simulink model "Inductance_Scan_model"  (R2022a)
settings: Solver=FixedStepAuto  StartTime=0.0  StopTime=.004  FixedStep=SampleTime  RelTol=1e-3
values from neighbouring files (symbols this model uses):
  Ad = sys_d_plasma.A    [All_injectors_LQG_bop_plasma_ss_model_code.m]    (also in All_injectors_LQG_bop_ss_model_code.m; All_injectors_LQG_continuous_time_code.m; All_injectors_LQG_plasma_7_15_24_code.m; All_injectors_LQG_plasma_ss_model_code.m)
  Amplitude = 600    [All_injectors_LQG_bop_plasma_ss_model_code.m]    (also in All_injectors_LQG_bop_ss_model_code.m; All_injectors_LQG_continuous_time_code.m; All_injectors_LQG_plasma_7_15_24_code.m; All_injectors_LQG_plasma_ss_model_code.m)
  Amplitude1 = 600    [All_injectors_vaccum.m]    (also in All_injectors_with_LQG_code.m; MPC_attempt.m; Plasma_ss_model.m; Use_for_freq_scan.m)
  Bd = sys_d_plasma.B    [All_injectors_LQG_bop_plasma_ss_model_code.m]    (also in All_injectors_LQG_bop_ss_model_code.m; All_injectors_LQG_continuous_time_code.m; All_injectors_LQG_plasma_7_15_24_code.m; All_injectors_LQG_plasma_ss_model_code.m)
  Cap = 96e-6    (= 9.6e-05)    [All_injectors_LQG_bop_ss_model_code.m]    (also in All_injectors_LQG_continuous_time_code.m; All_injectors_LQG_plasma_7_15_24_code.m; All_injectors_LQG_plasma_ss_model_code.m; All_injectors_vaccum.m)
  Cd = sys_d_plasma.C    [All_injectors_LQG_bop_plasma_ss_model_code.m]    (also in All_injectors_LQG_bop_ss_model_code.m; All_injectors_LQG_continuous_time_code.m; All_injectors_LQG_plasma_7_15_24_code.m; All_injectors_LQG_plasma_ss_model_code.m)
  Dd = sys_d_plasma.D    [All_injectors_LQG_bop_plasma_ss_model_code.m]    (also in All_injectors_LQG_bop_ss_model_code.m; All_injectors_LQG_continuous_time_code.m; All_injectors_LQG_plasma_7_15_24_code.m; All_injectors_LQG_plasma_ss_model_code.m)
  L1 = (9.78e-7)    (= 9.78e-07)    [All_injectors_LQG_bop_plasma_ss_model_code.m]    (also in All_injectors_LQG_bop_ss_model_code.m = 8.0141e-07; All_injectors_LQG_continuous_time_code.m = 8.0141e-07; All_injectors_LQG_plasma_7_15_24_code.m = 8.0141e-07; All_injectors_LQG_plasma_ss_model_code.m = 8.0141e-07)
  L2 = 2.0462e-6    (= 2.0462e-06)    [All_injectors_LQG_bop_ss_model_code.m]    (also in All_injectors_LQG_continuous_time_code.m; All_injectors_LQG_plasma_7_15_24_code.m; All_injectors_LQG_plasma_ss_model_code.m; All_injectors_vaccum.m = 9.3369e-07)
  Lp = L2    (= 2.0462e-06)    [All_injectors_LQG_bop_ss_model_code.m]    (also in All_injectors_LQG_continuous_time_code.m; All_injectors_LQG_plasma_7_15_24_code.m; All_injectors_LQG_plasma_ss_model_code.m; Plasma_ss_model.m = 1.0231e-06)
  M = .161*L2    (= 3.294382e-07)    [All_injectors_LQG_bop_ss_model_code.m]    (also in All_injectors_LQG_continuous_time_code.m; All_injectors_LQG_plasma_7_15_24_code.m; All_injectors_LQG_plasma_ss_model_code.m; All_injectors_vaccum.m = 1.5032409e-07)
  Mw = .1346*L2    (= 2.7541852e-07)    [All_injectors_LQG_bop_ss_model_code.m]    (also in All_injectors_LQG_continuous_time_code.m; All_injectors_LQG_plasma_7_15_24_code.m; All_injectors_LQG_plasma_ss_model_code.m; All_injectors_vaccum.m = 1.25674674e-07)
  NoisePower = 0    [All_injectors_LQG_bop_plasma_ss_model_code.m]    (also in All_injectors_LQG_bop_ss_model_code.m = 0.0001; All_injectors_LQG_continuous_time_code.m = 0.0001; All_injectors_LQG_plasma_7_15_24_code.m; All_injectors_LQG_plasma_ss_model_code.m = 0.0001)
  R = 1    [All_injectors_LQG_bop_plasma_ss_model_code.m]    (also in All_injectors_LQG_bop_ss_model_code.m = diag(1*ones(1,num_inputs)); All_injectors_LQG_continuous_time_code.m = diag(1*ones(1,num_inputs)); All_injectors_LQG_plasma_7_15_24_code.m = diag(1*ones(1,num_inputs)); All_injectors_LQG_plasma_ss_model_code.m = diag(1*ones(1,num_inputs)))
  R1 = .0025    (= 0.0025)    [All_injectors_LQG_bop_ss_model_code.m]    (also in All_injectors_LQG_continuous_time_code.m; All_injectors_LQG_plasma_7_15_24_code.m; All_injectors_LQG_plasma_ss_model_code.m; All_injectors_vaccum.m)
  R2 = .005    (= 0.005)    [All_injectors_LQG_bop_ss_model_code.m]    (also in All_injectors_LQG_continuous_time_code.m; All_injectors_LQG_plasma_7_15_24_code.m; All_injectors_LQG_plasma_ss_model_code.m; All_injectors_vaccum.m)
  R3 = .005    (= 0.005)    [All_injectors_LQG_bop_ss_model_code.m]    (also in All_injectors_LQG_continuous_time_code.m; All_injectors_LQG_plasma_7_15_24_code.m; All_injectors_LQG_plasma_ss_model_code.m; All_injectors_vaccum.m)
  RunTime = .004    (= 0.004)    [All_injectors_LQG_bop_plasma_ss_model_code.m]    (also in All_injectors_LQG_bop_ss_model_code.m; All_injectors_LQG_continuous_time_code.m; All_injectors_LQG_plasma_7_15_24_code.m; All_injectors_LQG_plasma_ss_model_code.m)
  SampleTime = 1e-7    (= 1e-07)    [All_injectors_LQG_bop_plasma_ss_model_code.m]    (also in All_injectors_LQG_bop_ss_model_code.m; All_injectors_LQG_continuous_time_code.m; All_injectors_LQG_plasma_7_15_24_code.m; All_injectors_LQG_plasma_ss_model_code.m)
  voltage = Amplitude*sin(2*pi*Frequency*time)    [All_injectors_LQG_bop_plasma_ss_model_code.m]    (also in All_injectors_LQG_bop_ss_model_code.m; All_injectors_LQG_continuous_time_code.m; All_injectors_LQG_plasma_7_15_24_code.m; All_injectors_LQG_plasma_ss_model_code.m)
undefined symbols (not defined in the file or in its folder): Discrete, L1_V, Time
libraries: spsSeriesRLCBranchLib x50, simulink x23, spsCurrentMeasurementLib x20, spsDCVoltageSourceLib x12, spsVoltageMeasurementLib x11, spsFullBridgeMMCExternalDCLinksLib x9, spsPWMGeneratorMultilevelLib x9, ctrlSharedLib x5, spsMosfetLib x4, spsParallelRLCBranchLib x2, spsMutualInductanceLib x1, spspowerguiLib x1
(part 2 of 2)

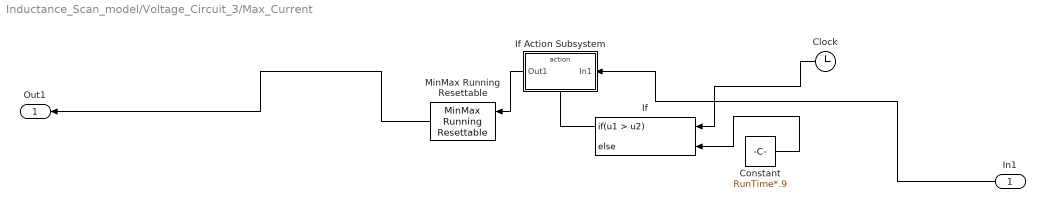
== system Inductance_Scan_model/Voltage_Circuit_3/Max_Current ==
  In1 : Inport
  Clock : Clock
  Constant : Constant  Value=RunTime*.9
  If : If  NumInputs=2  IfExpression=u1 > u2
  If Action Subsystem : Subsystem  TreatAsAtomicUnit=on
  MinMax Running Resettable : simulink/Math Operations/MinMax Running Resettable  Function=max  vinit=0.0
  Out1 : Outport
  wires:
  In1/1 -> If Action Subsystem/1(In1)
  If Action Subsystem/1(Out1) -> MinMax Running Resettable/1
  MinMax Running Resettable/1 -> Out1/1
  Constant/1 -> If/2
  Clock/1 -> If/1
  If/1 -> If Action Subsystem/Action

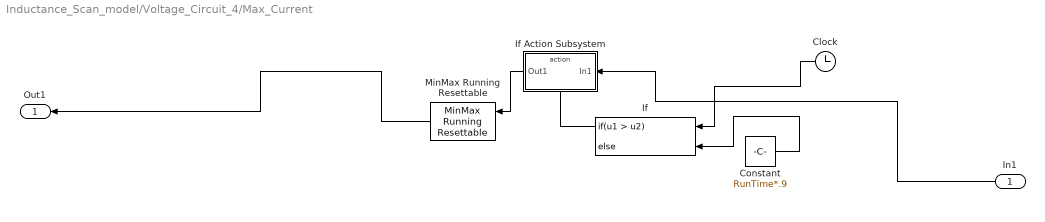
== system Inductance_Scan_model/Voltage_Circuit_4/Max_Current ==
  In1 : Inport
  Clock : Clock
  Constant : Constant  Value=RunTime*.9
  If : If  NumInputs=2  IfExpression=u1 > u2
  If Action Subsystem : Subsystem  TreatAsAtomicUnit=on
  MinMax Running Resettable : simulink/Math Operations/MinMax Running Resettable  Function=max  vinit=0.0
  Out1 : Outport
  wires:
  In1/1 -> If Action Subsystem/1(In1)
  If Action Subsystem/1(Out1) -> MinMax Running Resettable/1
  MinMax Running Resettable/1 -> Out1/1
  Constant/1 -> If/2
  Clock/1 -> If/1
  If/1 -> If Action Subsystem/Action

== system Inductance_Scan_model/Flux_Circuit_1/Max_Current/If Action Subsystem ==
  In1 : Inport
  Action Port : ActionPort  ActionPortLabel=if(u1 > u2)
  Out1 : Outport
  wires:
  In1/1 -> Out1/1

== system Inductance_Scan_model/Voltage_Circuit_1/Max_Current/If Action Subsystem ==
  In1 : Inport
  Action Port : ActionPort
  Out1 : Outport
  wires:
  In1/1 -> Out1/1

== system Inductance_Scan_model/Voltage_Circuit_2/Max_Current/If Action Subsystem ==
  In1 : Inport
  Action Port : ActionPort
  Out1 : Outport
  wires:
  In1/1 -> Out1/1

== system Inductance_Scan_model/Voltage_Circuit_3/Max_Current/If Action Subsystem ==
  In1 : Inport
  Action Port : ActionPort
  Out1 : Outport
  wires:
  In1/1 -> Out1/1

== system Inductance_Scan_model/Voltage_Circuit_4/Max_Current/If Action Subsystem ==
  In1 : Inport
  Action Port : ActionPort
  Out1 : Outport
  wires:
  In1/1 -> Out1/1
